simulink model "apcex4"  (Simulink 3.00)
settings: Solver=ode45  SolverMode=SingleTasking  StartTime=0.0  StopTime=4  RelTol=1e-3  AbsTol=1e-6

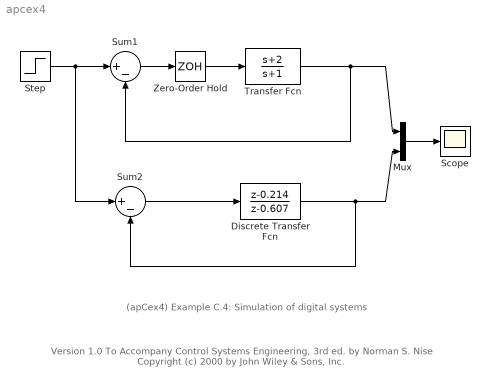
== system apcex4 ==
  note: (apCex4) Example C.4: Simulation of digital systems
  note: Version 1.0
      | To Accompany Control Systems Engineering, 3rd ed. by Norman S. Nise
      | Copyright (c) 2000 by John Wiley & Sons, Inc.
  Discrete Transfer Fcn : DiscreteTransferFcn  Numerator=[1 -0.214]  Denominator=[1 -0.607]  SampleTime=0.5
  Mux : Mux  Inputs=2
  Scope : Scope
      settings: TickLabels=on  TimeRange=auto  YMin=0  YMax=1  SaveToWorkspace=off  SaveName=ScopeData  DataFormat=Matrix
  Step : Step  Time=0  Before=0  After=1  SampleTime=-1
  Sum1 : Sum  Inputs=|+-  SaturateOnIntegerOverflow=on
  Sum2 : Sum  Inputs=|+-  SaturateOnIntegerOverflow=on
  Transfer Fcn : TransferFcn  Numerator=[1 2]  Denominator=[1 1]
  Zero-Order Hold : ZeroOrderHold  SampleTime=0.5
  wires:
  Zero-Order Hold/1 -> Transfer Fcn/1
  Sum1/1 -> Zero-Order Hold/1
  Sum2/1 -> Discrete Transfer Fcn/1
  Step/1 -> Sum1/1, Sum2/1
  Transfer Fcn/1 -> Sum1/2, Mux/1
  Discrete Transfer Fcn/1 -> Sum2/2, Mux/2
  Mux/1 -> Scope/1
